simulink model "expt_5_b"  (R2018b)
settings: Solver=VariableStepAuto  StartTime=0.0  StopTime=0.01  RelTol=1e-3
libraries: commanapbnd3 x1, commrandsrc3 x1
settings Model: Creator=sangh  LastModifiedBy=sangh

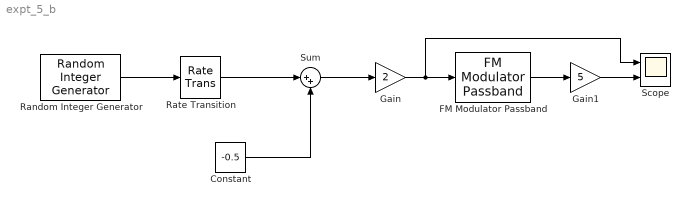
== system expt_5_b ==
  Constant : Constant  Value=-0.5
  FM Modulator Passband : commanapbnd3/FM Modulator Passband  Fc=10000  Ph=0  Kc=2000
      settings: SourceProductName=Communications System Toolbox  SourceProductBaseCode=CM
  Gain : Gain  Gain=2
  Gain1 : Gain  Gain=5
  Random Integer Generator : commrandsrc3/Random Integer Generator  SetSize=2  SeedSource=Auto  Seed=0  SampleTime=0.001  SamplesPerFrame=1  OutputDataType=boolean  SimulateUsing=Interpreted execution
  Rate Transition : RateTransition  OutPortSampleTime=2e-6
  Scope : Scope  NumInputPorts=2
  Sum : Sum  Inputs=|++
  wires:
  Random Integer Generator/1 -> Rate Transition/1
  Rate Transition/1 -> Sum/1
  Constant/1 -> Sum/2
  Sum/1 -> Gain/1
  Gain/1 -> Scope/1, FM Modulator Passband/1
  FM Modulator Passband/1 -> Gain1/1
  Gain1/1 -> Scope/2
